simulink model "FlexPWM_ISR"  (Simulink 8.1)
settings: Solver=FixedStepDiscrete  StartTime=0.0  StopTime=50.0  FixedStep=1.0  RelTol=1e-3
undefined symbols (not defined in the file or in its folder): A10, A14, B, B13, C6, D, L3, N3, P3, PA12, PA13, PD5, PD6, R10
libraries: rappid_564xl_ec_toolbox x6
settings Model: Creator=evarshavskaya  LastModifiedBy=evarshavskaya
settings DataIOCC: ExternalInput=off  InitialState=off  SaveOutput=off  SignalLogging=off  SaveTime=off
settings OptimizationCC: InlineParams=on  OptimizeModelRefInitCode=on  LifeSpan=1
settings DebuggingCC: InheritedTsInSrcMsg=none  SingleTaskRateTransMsg=error  UnconnectedInputMsg=error  UnconnectedOutputMsg=error  UnconnectedLineMsg=error  UnknownTsInhSupMsg=error
settings HardwareCC: ProdLargestAtomicInteger=Long  ProdLargestAtomicFloat=Double  ProdIntDivRoundTo=Zero  ProdEndianess=BigEndian  ProdHWDeviceType=Freescale->32-bit PowerPC
settings RTWCC: SystemTargetFile=rappid564xl.tlc  MakeCommand=rappid_564xl_make_rtw  TemplateMakefile=rappid_564xl_default_tmf  PostCodeGenCommand=rappid_analyzegencode(buildInfo)  Description=RAppID Toolbox MPC564xL Code Generation Target (rappid)  ProcessScript=rappid564xl_make_rtw_hook
settings CodeAppCC: IgnoreCustomStorageClasses=off  CustomSymbolStrType=$N$R$M  InternalIdentifier=Classic
settings STFCustomTargetCC: CodeReplacementLibrary=ANSI_C  ModelReferenceCompliant=off  CombineOutputUpdateFcns=on  SuppressErrorStatus=on  ERTCustomFileBanners=on  SupportContinuousTime=off  SupportNonInlinedSFcns=off  MATLABClassNameForMDSCustomization=Simulink.SoftwareTarget.ERTCustomization  GRTInterface=off  SystemTargetFile=rappid564xl.tlc
settings ERTTargetCC: CodeReplacementLibrary=ANSI_C  MultiwordLength=2048  ModelReferenceCompliant=off  ParMdlRefBuildCompliant=off  CompOptLevelCompliant=off  ConcurrentExecutionCompliant=off  SuppressErrorStatus=on  ERTFirstTimeCompliant=off  ModelStepFunctionPrototypeControlCompliant=off  CPPClassGenCompliant=off  ExtModeMexFile=noextcomm  InlinedParameterPlacement=NonHierarchical  ERTCustomFileTemplate=example_file_process.tlc  ConvertIfToSwitch=off  SuppressUnreachableDefaultCases=off

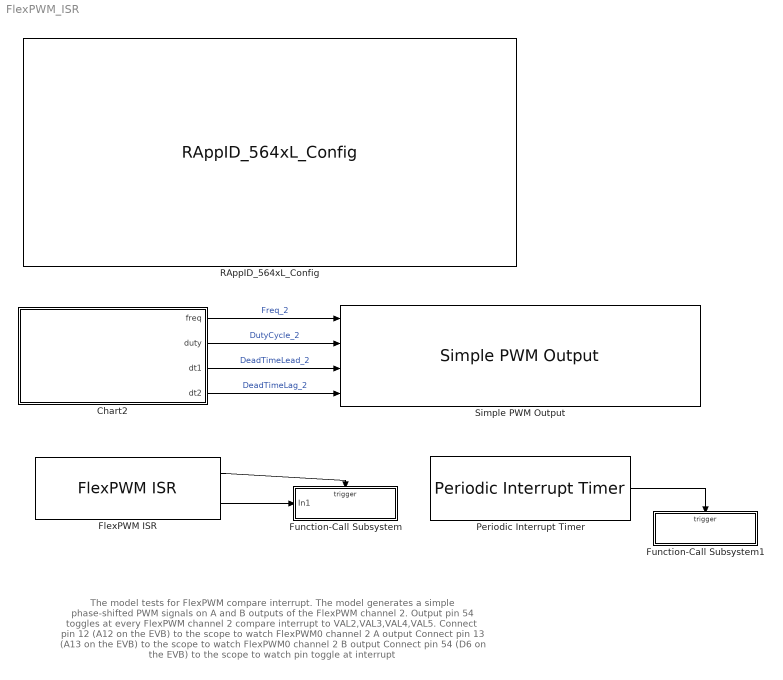
== system FlexPWM_ISR ==
  note: The model tests for FlexPWM compare interrupt.
      |
      | The model generates a simple phase-shifted PWM signals on A and B outputs of the FlexPWM channel 2.
      | Output pin 54 toggles at every FlexPWM channel 2 compare interrupt to VAL2,VAL3,VAL4,VAL5.
      |
      | Connect pin 12 (A12 on the EVB) to the scope to watch FlexPWM0 channel 2 A output
      | Connect pin 13 (A13 on the EVB) to the scope to watch FlexPWM0 channel 2 B output
      | Connect pin 54 (D6 on the EVB) to the scope to watch pin toggle at interrupt
  Chart2 : Stateflow chart  TreatAsAtomicUnit=on
  FlexPWM ISR : rappid_564xl_ec_toolbox/MPC564xL/Motor Control Blocks/FlexPWM ISR  Priority=2  intSource=Compare interrupt  intSrc=60  Module=0  pwmMod=0  SubModule=2  subMod=2  val0=off  val1=off  val2=on  val3=on  val4=on  val5=on  isrPriority=12  isrPrio=12  outMask=on
  Function-Call Subsystem : Subsystem  TreatAsAtomicUnit=on
      settings: RTWSystemCode=Nonreusable function
  Function-Call Subsystem1 : Subsystem  TreatAsAtomicUnit=on
      settings: RTWSystemCode=Nonreusable function
  Periodic Interrupt Timer : rappid_564xl_ec_toolbox/MPC564xL/General Purpose Blocks/Periodic Interrupt Timer  pit_chan=1  pit_timeout=50  int_priority=12  pit_timeout_val=5999999
  RAppID_564xL_Config : rappid_564xl_ec_toolbox/MPC564xL/RAppID_564xL_Config  SystemClock=120  XTAL=40  MC_clock_60=12  MC_clock_80=16  MC_clock_120=10  SWG_clock_60=20  SWG_clock_80=13.334  SWG_clock_120=20  Compiler=CodeWarrior  MemTarget=RAM  Part=MPC5643L  Package=144 LQFP  global_int_priority=10  base_tick_priority=14  sys_task_supress=off  exception_handlers=off  stored_mdl_name=FlexPWM_1  freemaster_interface=Oops  freemaster_rx_pin="LINFlex_0 Rx Pin 116 : \"PB[3]\""  freemaster_tx_pin="LINFlex_0 Tx Pin 114 : \"PB[2]\""  freemaster_interface_1=None  freemaster_enable=off  freemaster_rate=57600  freemaster_tx0_pin=18 : B[2] : 114 : A14  freemaster_rx0_pin=19 : B[3] : 116 : B13  freemaster_tx1_pin=57 : D[9] : 26 : L3  freemaster_rx1_pin=29 : B[13] : 60 : R10  freemaster_can_channel=1CH  freemater_can_speed=500K  freemaster_can_msgig=0x7AA  ccp_interface=None  ccp_enable=off  ccp_can_channel=CH1 (MB 0 - 1)  ccp_can_speed=500K  ccp_can_cro_id=256  ccp_can_dto_id=257  ccp_dev_id=RappID  ccp_dev_addr=0  ccp_odt=3  ccp_daq=3  pil_enable=off  pil_bam=on  comport=1  pil_rate=57600  bam_password_def=on  bam_password=0xFEEDFACECAFEBEEF  bam_sa_cs=off  bam_start_address=0x0  bam_code_size=0x7000  cons_dspi=on  cons_can=on  cons_adc=on  cons_pwm=on  cons_ctu=on  cons_swg=on  cons_eTimer=on  cons_fm=on
  Simple PWM Output : rappid_564xl_ec_toolbox/MPC564xL/Motor Control Blocks/Simple PWM Output  Priority=1  pwmModule=0  pwmMod=0  SubModule=2  subMod=2  InitFreq=1000  resolution=1 %  resValue=1  InitDutyA=60  InitDutyB=20  align=A - edge aligned B - phase shifted  PhaseShift_A=0  PhaseShift=30  Phase_A=0  Phase_B=30  centered=-1  DoubleS=off  doubleSw=off  debugSw=off  debug_mode=0  pin_A0=None  pin_B0=None  pin_X0=None  pin_A1=None  pin_B1=None  pin_X1=None  pin_A2="12  : PA12 : [ 122 ] : [ A10 ]"  pin_B2="13  : PA13 : [ 136 ] : [ C6 ]"  pin_X2=None  pin_A3=None  pin_B3=None  pin_X3=None  pin1_A0=None  pin1_B0=None  pin1_X0=None  pin1_A1=None  pin1_B1=None  pin1_X1=None  pin1_A2=None  pin1_B2=None  pin1_X2=None  pin1_A3=None  pin1_B3=None  pin1_X3=None  pcrNumA=12  pcrNumB=13  pcrNumX=255  polA=off  polB=off  polX=off  octrl=0  syncFrom0=off  masterSync=0  outVal0=off  outVal1=off  outVal2=on  outVal3=on  outVal4=on  outVal5=on  outTrig=60
  wires:
  Chart2/2(duty) -> Simple PWM Output/2  "DutyCycle_2"
  Chart2/3(dt1) -> Simple PWM Output/3  "DeadTimeLead_2"
  Chart2/4(dt2) -> Simple PWM Output/4  "DeadTimeLag_2"
  Chart2/1(freq) -> Simple PWM Output/1  "Freq_2"
  FlexPWM ISR/1 -> Function-Call Subsystem/Trigger
  FlexPWM ISR/2 -> Function-Call Subsystem/1(In1)
  Periodic Interrupt Timer/1 -> Function-Call Subsystem1/Trigger

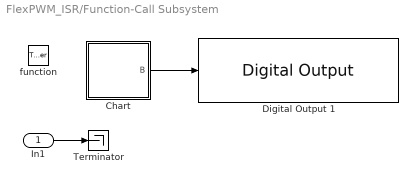
== system FlexPWM_ISR/Function-Call Subsystem ==
  In1 : Inport
  function : TriggerPort  TriggerType=function-call
  Chart : Stateflow chart  TreatAsAtomicUnit=on
  Digital Output 1 : rappid_564xl_ec_toolbox/MPC564xL/General Purpose Blocks/Digital Output   gpio_outputs="54  : PD6  : [ 34 ] : [ P3 ]"  pinNum=[ 34 ]  pcrNum=54
  Terminator : Terminator
  wires:
  In1/1 -> Terminator/1
  Chart/1(B) -> Digital Output 1/1

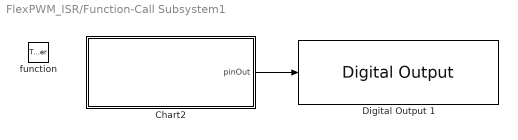
== system FlexPWM_ISR/Function-Call Subsystem1 ==
  function : TriggerPort  TriggerType=function-call
  Chart2 : Stateflow chart  TreatAsAtomicUnit=on
  Digital Output 1 : rappid_564xl_ec_toolbox/MPC564xL/General Purpose Blocks/Digital Output   gpio_outputs="53  : PD5  : [ 33 ] : [ N3 ]"  pinNum=[ 33 ]  pcrNum=53
  wires:
  Chart2/1(pinOut) -> Digital Output 1/1

== stateflow chart Chart2 ==
  settings: executeAtInitialization=1
  state A
    du:
    freq =2000;
    duty=60;
    dt1=20;
    dt2=30;
    cntr=cntr+1;
  state A1
    du:
    freq =2000;
    duty=40;
    dt1=30;
    dt2=60;
    cntr=cntr-1;
  (default) -> A : {cntr=0;}
  A1 -> A : [cntr < 2]
  A -> A1 : [cntr > 10]
  data: cntr local uint32 [0..1000] =0; freq output uint32 [0..10000]; duty output uint32 [0..100]; dt1 output uint32 [0..4095]; dt2 output uint32 [0..4095]

== stateflow chart Function-Call Subsystem/Chart ==
  state B
  state B1
  (default) -> B
  B -> B1
  B1 -> B
  data: B output boolean

== stateflow chart Function-Call Subsystem1/Chart2 ==
  settings: executeAtInitialization=1
  state A
    du:
    counter++;
    pinOut = 1;
  state A1
    du:
    counter--;
    pinOut = 0;
  (default) -> A : {counter=0;}
  A1 -> A : [counter < 0]
  A -> A1 : [counter > 5]
  data: counter local int16 =0; pinOut output boolean
